simulink model "nxtway_gs"  (Simulink 10.0)
settings: Solver=ode45  StartTime=0.0  StopTime=30  MaxStep=TS  RelTol=1e-3  EnableMultiTasking=on
PreLoadFcn:
  | param_nxtway_gs
undefined symbols (not defined in the file): BATTERY, D, GP_MAX, GYRO0, MAP_WALL, pwm_gain, pwm_offset, R, sigbuilder_block, START_POS, TIME_START, W
libraries: simulink x2
settings Model: Creator=y_yama  LastModifiedBy=bhisma
settings DataIOCC: SignalLoggingSaveFormat=ModelDataLogs  SaveOutput=off  SignalLogging=off  SaveTime=off
settings OptimizationCC: DefaultParameterBehavior=Inlined  InlineInvariantSignals=on  ExpressionDepthLimit=2147483647  InitFltsAndDblsToZero=on  LifeSpan=1
settings DebuggingCC: SolverPrmCheckMsg=warning  TasksWithSamePriorityMsg=none  SigSpecEnsureSampleTimeMsg=none  IntegerOverflowMsg=none  FcnCallInpInsideContextMsg=warning  UnknownTsInhSupMsg=none  StateNameClashWarn=warning  IntegerSaturationMsg=none
settings HardwareCC: ProdLargestAtomicInteger=Long  ProdLargestAtomicFloat=Float  ProdIntDivRoundTo=Zero  ProdEndianess=LittleEndian  ProdHWDeviceType=ARM Compatible->ARM 7
settings SFSimCC: SFSimEcho=off  SimUseLocalCustomCode=on  SimParseCustomCode=off  CustomCodeUndefinedFunction=FilterOut
settings RTWCC: RTWUseLocalCustomCode=on

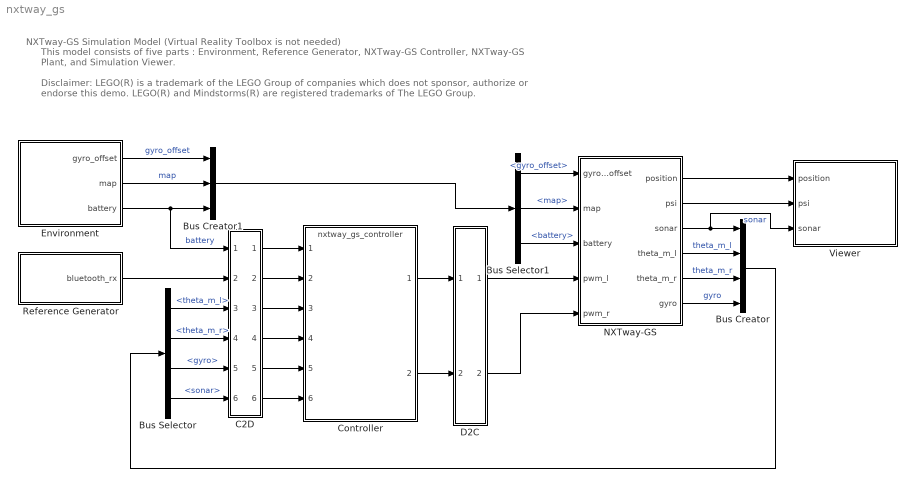
== system nxtway_gs ==
  note: Disclaimer:
      | LEGO(R) is a trademark of the LEGO Group of companies which does not sponsor, authorize or endorse this demo.
      | LEGO(R) and Mindstorms(R) are registered trademarks of The LEGO Group.
  note: NXTway-GS Simulation Model (Virtual Reality Toolbox is not needed)
  note: This model consists of five parts : Environment, Reference Generator, NXTway-GS Controller, NXTway-GS Plant, and Simulation Viewer.
  Bus Creator : BusCreator  Inputs=4
  Bus Creator1 : BusCreator  Inputs=3
  Bus Selector : BusSelector  OutputSignals=theta_m_l,theta_m_r,gyro,sonar
  Bus Selector1 : BusSelector  OutputSignals=gyro_offset,map,battery
  C2D : Subsystem
      mask Display: fprintf('C2D')
  Controller : ModelReference  ModelNameDialog=nxtway_gs_controller  SimulationMode=Normal  ModelReferenceVersion=1.721
  D2C : Subsystem
      mask Display: fprintf('D2C')
  Environment : Subsystem
  NXTway-GS : Subsystem
  Reference Generator : Subsystem
  Viewer : Subsystem
  wires:
  Bus Creator/1 -> Bus Selector/1
  Environment/3(battery) -> C2D/1(In1), Bus Creator1/3  "battery"
  Controller/1 -> D2C/1(In1)
  D2C/1(Out1) -> NXTway-GS/4(pwm_l)
  Controller/2 -> D2C/2(In2)
  D2C/2(Out2) -> NXTway-GS/5(pwm_r)
  C2D/1(Out1) -> Controller/1
  Reference Generator/1(bluetooth_rx) -> C2D/2(In2)
  C2D/2(Out2) -> Controller/2
  Bus Selector/1 -> C2D/3(In3)  "<theta_m_l>"
  Bus Selector/2 -> C2D/4(In4)  "<theta_m_r>"
  Bus Selector/3 -> C2D/5(In5)  "<gyro>"
  Bus Selector/4 -> C2D/6(In6)  "<sonar>"
  C2D/3(Out3) -> Controller/3
  C2D/4(Out4) -> Controller/4
  C2D/5(Out5) -> Controller/5
  C2D/6(Out6) -> Controller/6
  Environment/1(gyro_offset) -> Bus Creator1/1  "gyro_offset"
  Environment/2(map) -> Bus Creator1/2  "map"
  Bus Creator1/1 -> Bus Selector1/1
  Bus Selector1/1 -> NXTway-GS/1(gyro_offset)  "<gyro_offset>"
  Bus Selector1/2 -> NXTway-GS/2(map)  "<map>"
  Bus Selector1/3 -> NXTway-GS/3(battery)  "<battery>"
  NXTway-GS/2(psi) -> Viewer/2(psi)
  NXTway-GS/1(position) -> Viewer/1(position)
  NXTway-GS/3(sonar) -> Bus Creator/1, Viewer/3(sonar)  "sonar"
  NXTway-GS/4(theta_m_l) -> Bus Creator/2  "theta_m_l"
  NXTway-GS/5(theta_m_r) -> Bus Creator/3  "theta_m_r"
  NXTway-GS/6(gyro) -> Bus Creator/4  "gyro"

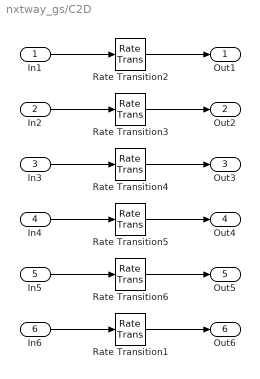
== system nxtway_gs/C2D ==
  In1 : Inport
  In2 : Inport  Port=2
  In3 : Inport  Port=3
  In4 : Inport  Port=4
  In5 : Inport  Port=5
  In6 : Inport  Port=6
  Rate Transition{1..6} (6 alike) : RateTransition  Integrity=off  OutPortSampleTime=TS
      settings: AttributesFormatString=Ts=%<OutPortSampleTime>
  Out1 : Outport
  Out2 : Outport  Port=2
  Out3 : Outport  Port=3
  Out4 : Outport  Port=4
  Out5 : Outport  Port=5
  Out6 : Outport  Port=6
  wires:
  In1/1 -> Rate Transition2/1
  Rate Transition2/1 -> Out1/1
  In2/1 -> Rate Transition3/1
  In3/1 -> Rate Transition4/1
  Rate Transition3/1 -> Out2/1
  Rate Transition4/1 -> Out3/1
  In4/1 -> Rate Transition5/1
  Rate Transition5/1 -> Out4/1
  In5/1 -> Rate Transition6/1
  Rate Transition6/1 -> Out5/1
  In6/1 -> Rate Transition1/1
  Rate Transition1/1 -> Out6/1

== system nxtway_gs/D2C ==
  In1 : Inport
  In2 : Inport  Port=2
  Rate Transition : RateTransition  Integrity=off  OutPortSampleTime=0
      settings: AttributesFormatString=Ts=%<OutPortSampleTime>
  Rate Transition1 : RateTransition  Integrity=off  OutPortSampleTime=0
      settings: AttributesFormatString=Ts=%<OutPortSampleTime>
  Out1 : Outport  SampleTime=0
  Out2 : Outport  Port=2  SampleTime=0
  wires:
  Rate Transition/1 -> Out1/1
  In1/1 -> Rate Transition/1
  Rate Transition1/1 -> Out2/1
  In2/1 -> Rate Transition1/1

== system nxtway_gs/Environment ==
  note: Environment
  note: The charactaristics of sensors of NXTway-GS and external environment.
  Constant : Constant  Value=GYRO0  OutDataTypeStr=uint16
      settings: AttributesFormatString=DataType = %<OutDataTypeStr>
  Constant1 : Constant  Value=MAP_WALL  VectorParams1D=off  OutDataTypeStr=boolean
      settings: AttributesFormatString=DataType = %<OutDataTypeStr>
  Constant2 : Constant  Value=BATTERY  OutDataTypeStr=uint16
      settings: AttributesFormatString=DataType = %<OutDataTypeStr>
  gyro_offset : Outport
  map : Outport  Port=2
  battery : Outport  Port=3
  wires:
  Constant1/1 -> map/1
  Constant/1 -> gyro_offset/1
  Constant2/1 -> battery/1

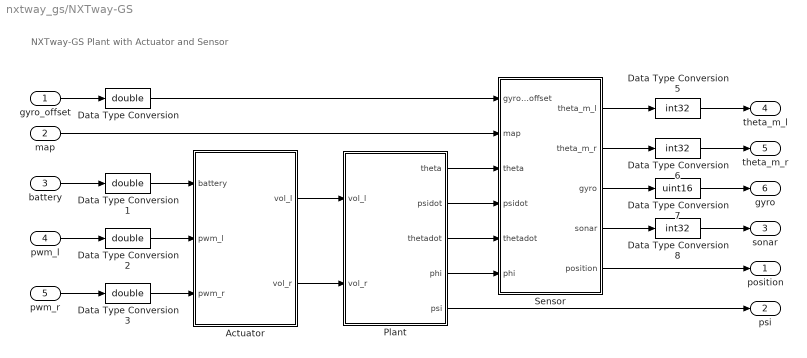
== system nxtway_gs/NXTway-GS ==
  note: NXTway-GS Plant with Actuator and Sensor
  gyro_offset : Inport
  map : Inport  Port=2
  battery : Inport  Port=3
  pwm_l : Inport  Port=4
  pwm_r : Inport  Port=5
  Actuator : Subsystem
  Data Type Conversion{,1..3} (4 alike) : DataTypeConversion  OutDataTypeStr=double  RndMeth=Nearest
      settings: AttributesFormatString=Round = %<RndMeth>
  Data Type Conversion5 : DataTypeConversion  OutDataTypeStr=int32  RndMeth=Nearest
      settings: AttributesFormatString=Round = %<RndMeth>
  Data Type Conversion6 : DataTypeConversion  OutDataTypeStr=int32  RndMeth=Nearest
      settings: AttributesFormatString=Round = %<RndMeth>
  Data Type Conversion7 : DataTypeConversion  OutDataTypeStr=uint16  RndMeth=Nearest
      settings: AttributesFormatString=Round = %<RndMeth>
  Data Type Conversion8 : DataTypeConversion  OutDataTypeStr=int32  RndMeth=Nearest
      settings: AttributesFormatString=Round = %<RndMeth>
  Plant : Subsystem
  Sensor : Subsystem
  position : Outport
  psi : Outport  Port=2
  sonar : Outport  Port=3
  theta_m_l : Outport  Port=4
  theta_m_r : Outport  Port=5
  gyro : Outport  Port=6
  wires:
  Actuator/1(vol_l) -> Plant/1(vol_l)
  Actuator/2(vol_r) -> Plant/2(vol_r)
  Plant/2(psidot) -> Sensor/4(psidot)
  Plant/1(theta) -> Sensor/3(theta)
  battery/1 -> Data Type Conversion1/1
  gyro_offset/1 -> Data Type Conversion/1
  map/1 -> Sensor/2(map)
  Sensor/1(theta_m_l) -> Data Type Conversion5/1
  Sensor/2(theta_m_r) -> Data Type Conversion6/1
  pwm_l/1 -> Data Type Conversion2/1
  Sensor/3(gyro) -> Data Type Conversion7/1
  Plant/3(thetadot) -> Sensor/5(thetadot)
  Sensor/4(sonar) -> Data Type Conversion8/1
  pwm_r/1 -> Data Type Conversion3/1
  Plant/5(psi) -> psi/1
  Data Type Conversion/1 -> Sensor/1(gyro_offset)
  Data Type Conversion1/1 -> Actuator/1(battery)
  Data Type Conversion2/1 -> Actuator/2(pwm_l)
  Data Type Conversion3/1 -> Actuator/3(pwm_r)
  Data Type Conversion5/1 -> theta_m_l/1
  Data Type Conversion6/1 -> theta_m_r/1
  Data Type Conversion7/1 -> gyro/1
  Sensor/5(position) -> position/1
  Plant/4(phi) -> Sensor/6(phi)
  Data Type Conversion8/1 -> sonar/1

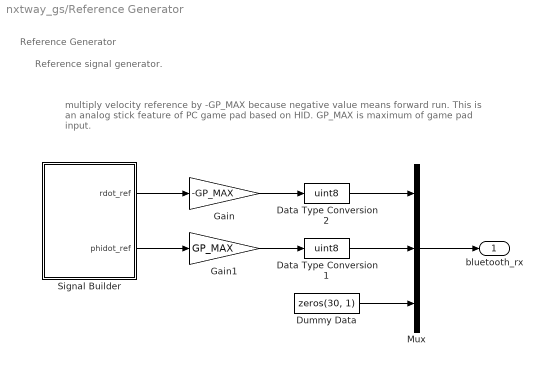
== system nxtway_gs/Reference Generator ==
  note: Reference Generator
  note: Reference signal generator.
  note: multiply velocity reference by -GP_MAX because negative value
      | means forward run. This is an analog stick feature of PC game pad
      | based on HID. GP_MAX is maximum of game pad input.
  Data Type Conversion1 : DataTypeConversion  OutDataTypeStr=uint8  RndMeth=Nearest
      settings: AttributesFormatString=Round = %<RndMeth>
  Data Type Conversion2 : DataTypeConversion  OutDataTypeStr=uint8  RndMeth=Nearest
      settings: AttributesFormatString=Round = %<RndMeth>
  Dummy Data : Constant  Value=zeros(30, 1)  OutDataTypeStr=uint8
      settings: AttributesFormatString=DataType = %<OutDataTypeStr>
  Gain : Gain  Gain=-GP_MAX  OutDataTypeStr=Inherit: Same as input  ParamDataTypeStr=Inherit: Same as input
  Gain1 : Gain  Gain=GP_MAX  OutDataTypeStr=Inherit: Same as input  ParamDataTypeStr=Inherit: Same as input
  Mux : Mux  Inputs=3
  Signal Builder : Subsystem  Tag=STV Subsys  LoadFcn=sigbuilder_block('load');  StartFcn=sigbuilder_block('start');  StopFcn=sigbuilder_block('stop');  ClipboardFcn=sigbuilder_block('clipboard');  mask(Sigbuilder block){tuvar=[0:10]}
      mask help: Sigbuilder GUI
      mask init:
      | if ~strcmp(get_param(bdroot(gcbh),'SimulationStatus'),'stopped') tuvar = sigbuilder_block('maskInit'); end
      settings: CopyFcn=sigbuilder_block('copy');  DeleteFcn=sigbuilder_block('delete');  ModelCloseFcn=sigbuilder_block('modelClose');  PreSaveFcn=sigbuilder_block('preSave');  PauseFcn=sigbuilder_block('pause')  ContinueFcn=sigbuilder_block('continue')  NameChangeFcn=sigbuilder_block('namechange');  OpenFcn=sigbuilder_block('open',[103.5 117.75 516 349.5 ]);  CloseFcn=sigbuilder_block('close');
      mask Display: plot(0, 0, 100, 100,[2, 2, 32, 32, 2], [68, 8, 8, 68, 68],[32, 2], [38, 38], [32, 19, 2],[53, 60, 44], [32, 17, 17, 2],[16, 16, 31, 31]);txt = getActiveGroup(gcbh);text(2, 100, txt,'verticalAlignment', 'top');
  bluetooth_rx : Outport
  wires:
  Data Type Conversion2/1 -> Mux/1
  Data Type Conversion1/1 -> Mux/2
  Dummy Data/1 -> Mux/3
  Mux/1 -> bluetooth_rx/1
  Signal Builder/1(rdot_ref) -> Gain/1
  Gain/1 -> Data Type Conversion2/1
  Gain1/1 -> Data Type Conversion1/1
  Signal Builder/2(phidot_ref) -> Gain1/1

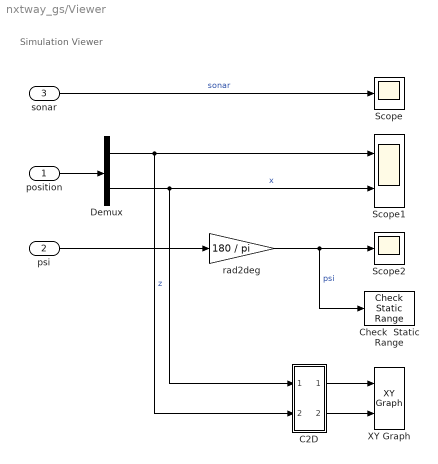
== system nxtway_gs/Viewer ==
  note: Simulation Viewer
  position : Inport
  psi : Inport  Port=2
  sonar : Inport  Port=3
  C2D : Subsystem
      mask Display: fprintf('C2D')
  Check  Static Range : simulink/Model Verification/Check  Static Range  Description=BODY_ANGLE_MIN <= u <= BODY_ANGLE_MAX  max=BODY_ANGLE_MAX  max_included=on  min=BODY_ANGLE_MIN  min_included=on  enabled=on  stopWhenAssertionFail=on  export=off  icon=graphic
      settings: SourceProductName=Simulink  SourceProductBaseCode=SL
  Demux : Demux  Outputs=2
  Scope : Scope
  Scope1 : Scope  NumInputPorts=2
  Scope2 : Scope
  XY Graph : simulink/Sinks/XY Graph  xmin=-100  xmax=300  ymin=-100  ymax=300  st=-1
  rad2deg : Gain  Gain=180 / pi
  wires:
  rad2deg/1 -> Check  Static Range/1, Scope2/1  "psi"
  Demux/1 -> Scope1/1, C2D/2(In2)  "z"
  Demux/2 -> Scope1/2, C2D/1(In1)  "x"
  psi/1 -> rad2deg/1
  sonar/1 -> Scope/1  "sonar"
  position/1 -> Demux/1
  C2D/1(Out1) -> XY Graph/1
  C2D/2(Out2) -> XY Graph/2

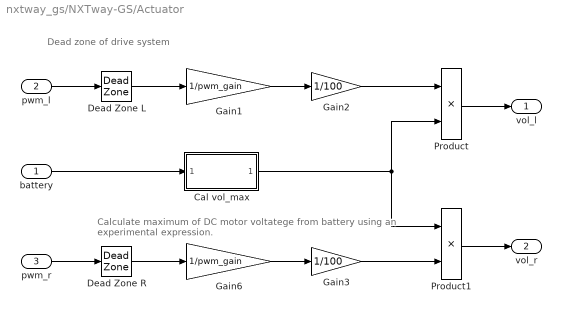
== system nxtway_gs/NXTway-GS/Actuator ==
  note: Dead zone of drive system
  note: Calculate maximum of DC motor voltatege from
      | battery using an experimental expression.
  battery : Inport
  pwm_l : Inport  Port=2
  pwm_r : Inport  Port=3
  Cal vol_max : Subsystem
  Dead Zone L : DeadZone  LowerValue=-pwm_offset  UpperValue=pwm_offset  SaturateOnIntegerOverflow=on
      settings: AttributesFormatString=start=%<LowerValue>\nend=%<UpperValue>
  Dead Zone R : DeadZone  LowerValue=-pwm_offset  UpperValue=pwm_offset  SaturateOnIntegerOverflow=on
      settings: AttributesFormatString=start=%<LowerValue>\nend=%<UpperValue>
  Gain1 : Gain  Gain=1/pwm_gain  OutDataTypeStr=Inherit: Same as input  ParamDataTypeStr=Inherit: Same as input
  Gain2 : Gain  Gain=1/100  OutDataTypeStr=Inherit: Same as input  ParamDataTypeStr=Inherit: Same as input
  Gain3 : Gain  Gain=1/100  OutDataTypeStr=Inherit: Same as input  ParamDataTypeStr=Inherit: Same as input
  Gain6 : Gain  Gain=1/pwm_gain  OutDataTypeStr=Inherit: Same as input  ParamDataTypeStr=Inherit: Same as input
  Product : Product  RndMeth=Simplest
  Product1 : Product  RndMeth=Simplest
  vol_l : Outport
  vol_r : Outport  Port=2
  wires:
  pwm_l/1 -> Dead Zone L/1
  pwm_r/1 -> Dead Zone R/1
  Gain1/1 -> Gain2/1
  Gain6/1 -> Gain3/1
  Gain2/1 -> Product/1
  Product/1 -> vol_l/1
  Gain3/1 -> Product1/2
  Product1/1 -> vol_r/1
  Dead Zone L/1 -> Gain1/1
  Dead Zone R/1 -> Gain6/1
  Cal vol_max/1(vol_max) -> Product/2, Product1/1
  battery/1 -> Cal vol_max/1(battery)

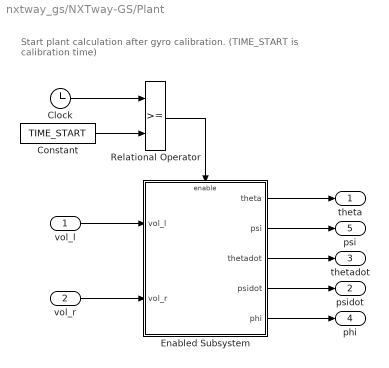
== system nxtway_gs/NXTway-GS/Plant ==
  note: Start plant calculation after gyro calibration.
      | (TIME_START is calibration time)
  vol_l : Inport
  vol_r : Inport  Port=2
  Clock : Clock
  Constant : Constant  Value=TIME_START  OutDataTypeStr=double
      settings: AttributesFormatString=DataType = %<OutDataTypeStr>
  Enabled Subsystem : Subsystem  TreatAsAtomicUnit=on
  Relational Operator : RelationalOperator  OutDataTypeStr=boolean  RndMeth=Nearest
  theta : Outport
  psidot : Outport  Port=2
  thetadot : Outport  Port=3
  phi : Outport  Port=4
  psi : Outport  Port=5
  wires:
  vol_l/1 -> Enabled Subsystem/1(vol_l)
  vol_r/1 -> Enabled Subsystem/2(vol_r)
  Relational Operator/1 -> Enabled Subsystem/Enable
  Clock/1 -> Relational Operator/1
  Constant/1 -> Relational Operator/2
  Enabled Subsystem/1(theta) -> theta/1
  Enabled Subsystem/3(thetadot) -> thetadot/1
  Enabled Subsystem/2(psi) -> psi/1
  Enabled Subsystem/5(phi) -> phi/1
  Enabled Subsystem/4(psidot) -> psidot/1

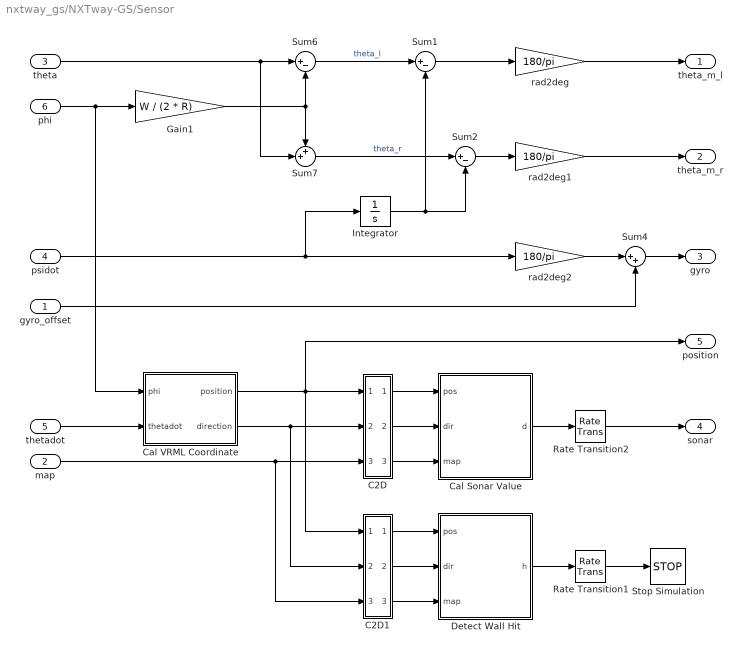
== system nxtway_gs/NXTway-GS/Sensor ==
  gyro_offset : Inport
  map : Inport  Port=2
  theta : Inport  Port=3
  psidot : Inport  Port=4
  thetadot : Inport  Port=5
  phi : Inport  Port=6
  C2D : Subsystem
      mask Display: fprintf('C2D')
  C2D1 : Subsystem
      mask Display: fprintf('C2D')
  Cal Sonar Value : MATLAB Function  TreatAsAtomicUnit=on
  Cal VRML Coordinate : Subsystem
  Detect Wall Hit : MATLAB Function  TreatAsAtomicUnit=on
  Gain1 : Gain  Gain=W / (2 * R)
  Integrator : Integrator
  Rate Transition1 : RateTransition  Integrity=off  OutPortSampleTime=0
      settings: AttributesFormatString=Ts=%<OutPortSampleTime>
  Rate Transition2 : RateTransition  Integrity=off  OutPortSampleTime=0
      settings: AttributesFormatString=Ts=%<OutPortSampleTime>
  Stop Simulation : Stop
  Sum1 : Sum  Inputs=|+-
  Sum2 : Sum  Inputs=|+-
  Sum4 : Sum  Inputs=|++
  Sum6 : Sum  Inputs=|+-
  Sum7 : Sum  Inputs=++|
  rad2deg : Gain  Gain=180/pi
  rad2deg1 : Gain  Gain=180/pi
  rad2deg2 : Gain  Gain=180/pi
  theta_m_l : Outport
  theta_m_r : Outport  Port=2
  gyro : Outport  Port=3
  sonar : Outport  Port=4
  position : Outport  Port=5
  wires:
  Integrator/1 -> Sum2/2, Sum1/2
  Sum4/1 -> gyro/1
  gyro_offset/1 -> Sum4/2
  Sum7/1 -> Sum2/1  "theta_r"
  rad2deg2/1 -> Sum4/1
  theta/1 -> Sum7/2, Sum6/1
  phi/1 -> Gain1/1, Cal VRML Coordinate/1(phi)
  Gain1/1 -> Sum7/1, Sum6/2
  Sum1/1 -> rad2deg/1
  psidot/1 -> Integrator/1, rad2deg2/1
  Sum2/1 -> rad2deg1/1
  rad2deg/1 -> theta_m_l/1
  rad2deg1/1 -> theta_m_r/1
  Sum6/1 -> Sum1/1  "theta_l"
  thetadot/1 -> Cal VRML Coordinate/2(thetadot)
  Cal Sonar Value/1(d) -> Rate Transition2/1
  Rate Transition2/1 -> sonar/1
  Cal VRML Coordinate/1(position) -> position/1, C2D/1(In1), C2D1/1(In1)
  map/1 -> C2D1/3(In3), C2D/3(In3)
  C2D/3(Out3) -> Cal Sonar Value/3(map)
  C2D/1(Out1) -> Cal Sonar Value/1(pos)
  Cal VRML Coordinate/2(direction) -> C2D/2(In2), C2D1/2(In2)
  C2D/2(Out2) -> Cal Sonar Value/2(dir)
  Detect Wall Hit/1(h) -> Rate Transition1/1
  C2D1/1(Out1) -> Detect Wall Hit/1(pos)
  C2D1/2(Out2) -> Detect Wall Hit/2(dir)
  C2D1/3(Out3) -> Detect Wall Hit/3(map)
  Rate Transition1/1 -> Stop Simulation/1

== system nxtway_gs/Reference Generator/Signal Builder ==
  Demux : Demux  Tag=STV Demux  Outputs=2
  FromWs : FromWorkspace  Tag=STV FromWs  VariableName=tuvar  SampleTime=0  SigBuilderData=DataTag0  VnvData=DataTag1
      SigBuilderData=|
      | common.afterFinalStr = 'Extrapolate'
      | common.sampleTime = 0
      | dataSet(1).timeRange = [0 25]
      | dataSet(1).name = 'Stand'
      | dataSet(2).timeRange = [0 25]
      | dataSet(2).name = 'Forward & Back'
      | dataSet(3).timeRange = [0 25]
      | dataSet(3).name = 'Turn'
      | dataSet(4).timeRange = [0 25]
      | dataSet(4).name = 'Approach Wall'
      | sbobj.Groups(1).Name = 'Stand'
      | sbobj.Groups(1).Signals(1).Name = 'rdot_ref'
      | sbobj.Groups(1).Signals(1).XData = [0 25]
      | sbobj.Groups(1).Signals(1).YData = [0 0]
      | sbobj.Groups(1).Signals(2).Name = 'phidot_ref'
      | sbobj.Groups(1).Signals(2).XData = [0 25]
      | sbobj.Groups(1).Signals(2).YData = [0 0]
      | sbobj.Groups(1).TimeRange = [0 25]
      | sbobj.Groups(2).Name = 'Forward & Back'
      | sbobj.Groups(2).Signals(1).Name = 'rdot_ref'
      | sbobj.Groups(2).Signals(1).XData = [0 5 5 10 10 15 15 20 20 25]
      | sbobj.Groups(2).Signals(1).YData = [0 0 1 1 0 0 -1 -1 0 0]
      | sbobj.Groups(2).Signals(2).Name = 'phidot_ref'
      | sbobj.Groups(2).Signals(2).XData = [0 25]
      | sbobj.Groups(2).Signals(2).YData = [0 0]
      | sbobj.Groups(2).TimeRange = [0 25]
      | sbobj.Groups(3).Name = 'Turn'
      | sbobj.Groups(3).Signals(1).Name = 'rdot_ref'
      | sbobj.Groups(3).Signals(1).XData = [0 10 10 15 15 20 20 25]
      | sbobj.Groups(3).Signals(1).YData = [0 0 1 1 0 0 1 1]
      | sbobj.Groups(3).Signals(2).Name = 'phidot_ref'
      | sbobj.Groups(3).Signals(2).XData = [0 5 5 10 10 15 15 20 20 25]
      | sbobj.Groups(3).Signals(2).YData = [0 0 1 1 0 0 -1 -1 0 0]
      | sbobj.Groups(3).TimeRange = [0 25]
      | sbobj.Groups(4).Name = 'Approach Wall'
      | sbobj.Groups(4).Signals(1).Name = 'rdot_ref'
      | sbobj.Groups(4).Signals(1).XData = [0 6.4 6.4 25]
      | sbobj.Groups(4).Signals(1).YData = [0 0 1 1]
      | sbobj.Groups(4).Signals(2).Name = 'phidot_ref'
      | sbobj.Groups(4).Signals(2).XData = [0 5 5 6.4 6.4 15 20 25]
      | sbobj.Groups(4).Signals(2).YData = [0 0 -1 -1 0 0 0 0]
      | sbobj.Groups(4).TimeRange = [0 25]
  rdot_ref : Outport  Tag=STV Outport
  phidot_ref : Outport  Tag=STV Outport  Port=2
  wires:
  FromWs/1 -> Demux/1
  Demux/1 -> rdot_ref/1
  Demux/2 -> phidot_ref/1

== system nxtway_gs/Viewer/C2D ==
  In1 : Inport
  In2 : Inport  Port=2
  Rate Transition1 : RateTransition  Integrity=off  OutPortSampleTime=TS_VR
      settings: AttributesFormatString=Ts=%<OutPortSampleTime>
  Rate Transition2 : RateTransition  Integrity=off  OutPortSampleTime=TS_VR
      settings: AttributesFormatString=Ts=%<OutPortSampleTime>
  Out1 : Outport
  Out2 : Outport  Port=2
  wires:
  Rate Transition1/1 -> Out2/1
  In2/1 -> Rate Transition1/1
  Rate Transition2/1 -> Out1/1
  In1/1 -> Rate Transition2/1

== system nxtway_gs/NXTway-GS/Actuator/Cal vol_max ==
  battery : Inport
  Constant : Constant  Value=0.625  OutDataTypeStr=double
      settings: AttributesFormatString=DataType = %<OutDataTypeStr>
  Gain3 : Gain  Gain=0.001089  OutDataTypeStr=Inherit: Same as input  ParamDataTypeStr=Inherit: Same as input
  Sum2 : Sum  Inputs=|+-  OutDataTypeStr=Inherit: Same as first input
  vol_max : Outport
  wires:
  battery/1 -> Gain3/1
  Gain3/1 -> Sum2/1
  Sum2/1 -> vol_max/1
  Constant/1 -> Sum2/2

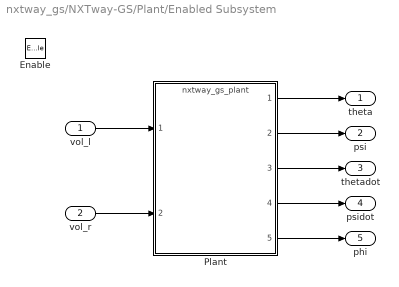
== system nxtway_gs/NXTway-GS/Plant/Enabled Subsystem ==
  vol_l : Inport
  vol_r : Inport  Port=2
  Enable : EnablePort
  Plant : ModelReference  ModelNameDialog=nxtway_gs_plant  SimulationMode=Normal  ModelReferenceVersion=1.41
  theta : Outport  InitialOutput=0
  psi : Outport  Port=2  InitialOutput=0
  thetadot : Outport  Port=3  InitialOutput=0
  psidot : Outport  Port=4  InitialOutput=0
  phi : Outport  Port=5  InitialOutput=0
  wires:
  vol_l/1 -> Plant/1
  vol_r/1 -> Plant/2
  Plant/1 -> theta/1
  Plant/2 -> psi/1
  Plant/3 -> thetadot/1
  Plant/4 -> psidot/1
  Plant/5 -> phi/1

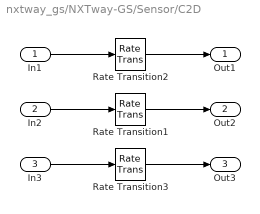
== system nxtway_gs/NXTway-GS/Sensor/C2D ==
  In1 : Inport
  In2 : Inport  Port=2
  In3 : Inport  Port=3
  Rate Transition1 : RateTransition  Integrity=off  OutPortSampleTime=TS_SONAR
      settings: AttributesFormatString=Ts=%<OutPortSampleTime>
  Rate Transition2 : RateTransition  Integrity=off  OutPortSampleTime=TS_SONAR
      settings: AttributesFormatString=Ts=%<OutPortSampleTime>
  Rate Transition3 : RateTransition  Integrity=off  OutPortSampleTime=TS_SONAR
      settings: AttributesFormatString=Ts=%<OutPortSampleTime>
  Out1 : Outport
  Out2 : Outport  Port=2
  Out3 : Outport  Port=3
  wires:
  Rate Transition3/1 -> Out3/1
  Rate Transition1/1 -> Out2/1
  In3/1 -> Rate Transition3/1
  In2/1 -> Rate Transition1/1
  Rate Transition2/1 -> Out1/1
  In1/1 -> Rate Transition2/1

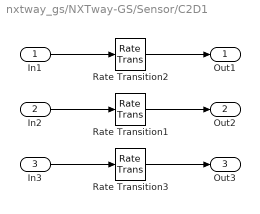
== system nxtway_gs/NXTway-GS/Sensor/C2D1 ==
  In1 : Inport
  In2 : Inport  Port=2
  In3 : Inport  Port=3
  Rate Transition1 : RateTransition  Integrity=off  OutPortSampleTime=TS_WALL
      settings: AttributesFormatString=Ts=%<OutPortSampleTime>
  Rate Transition2 : RateTransition  Integrity=off  OutPortSampleTime=TS_WALL
      settings: AttributesFormatString=Ts=%<OutPortSampleTime>
  Rate Transition3 : RateTransition  Integrity=off  OutPortSampleTime=TS_WALL
      settings: AttributesFormatString=Ts=%<OutPortSampleTime>
  Out1 : Outport
  Out2 : Outport  Port=2
  Out3 : Outport  Port=3
  wires:
  In1/1 -> Rate Transition2/1
  Rate Transition2/1 -> Out1/1
  In2/1 -> Rate Transition1/1
  In3/1 -> Rate Transition3/1
  Rate Transition1/1 -> Out2/1
  Rate Transition3/1 -> Out3/1

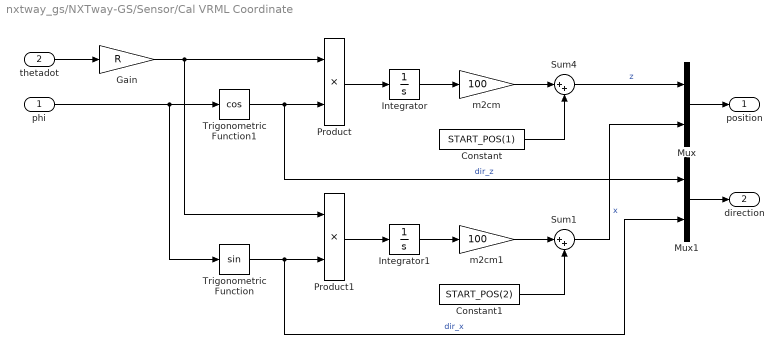
== system nxtway_gs/NXTway-GS/Sensor/Cal VRML Coordinate ==
  phi : Inport
  thetadot : Inport  Port=2
  Constant : Constant  Value=START_POS(1)  OutDataTypeStr=double
      settings: AttributesFormatString=DataType = %<OutDataTypeStr>
  Constant1 : Constant  Value=START_POS(2)  OutDataTypeStr=double
      settings: AttributesFormatString=DataType = %<OutDataTypeStr>
  Gain : Gain  Gain=R
  Integrator : Integrator
  Integrator1 : Integrator
  Mux : Mux  Inputs=2
  Mux1 : Mux  Inputs=2
  Product : Product  RndMeth=Simplest
  Product1 : Product  RndMeth=Simplest
  Sum1 : Sum  Inputs=|++
  Sum4 : Sum  Inputs=|++
  Trigonometric Function : Trigonometry
  Trigonometric Function1 : Trigonometry  Operator=cos
  m2cm : Gain  Gain=100
  m2cm1 : Gain  Gain=100
  position : Outport
  direction : Outport  Port=2
  wires:
  Product1/1 -> Integrator1/1
  Trigonometric Function/1 -> Product1/2, Mux1/2  "dir_x"
  Product/1 -> Integrator/1
  Trigonometric Function1/1 -> Product/2, Mux1/1  "dir_z"
  thetadot/1 -> Gain/1
  phi/1 -> Trigonometric Function1/1, Trigonometric Function/1
  Integrator/1 -> m2cm/1
  Integrator1/1 -> m2cm1/1
  Gain/1 -> Product1/1, Product/1
  m2cm/1 -> Sum4/1
  Sum4/1 -> Mux/1  "z"
  Constant/1 -> Sum4/2
  m2cm1/1 -> Sum1/1
  Constant1/1 -> Sum1/2
  Sum1/1 -> Mux/2  "x"
  Mux/1 -> position/1
  Mux1/1 -> direction/1

== matlab function NXTway-GS/Sensor/Detect Wall Hit ==
  data: pos input double; h output boolean; dir input double; map input double; D parameter double; W parameter double
function h = hit_wall(pos, dir, map, D, W)
% Detect if NXTway hits the wall
% Inputs:
%   pos    : NXTway position ([z, x]) [cm]
%   dir    : NXTway direction vector ([z, x]) [cm]
%   map    : wall map
% Outputs:
%   h      : wall hit flag

eml.extrinsic('errordlg');

h = false;
posh = zeros(6, 2);
[rows, cols] = size(map);
tmp1 = (D / 2) * dir;
tmp2 = (W / 2) * [dir(2), -dir(1)];

posh(2, :) = pos + tmp1;
posh(5, :) = pos - tmp1;
posh(1, :) = posh(2, :) + tmp2;
posh(6, :) = posh(5, :) + tmp2;
posh(3, :) = posh(2, :) - tmp2;
posh(4, :) = posh(5, :) - tmp2;

for n = 1:6
	if posh(n, 1) <= 0 || posh(n, 1) >= rows ...
			|| posh(n, 2) <= 0 || posh(n, 2) >= cols
		% outside map
		h = false;
	else
		% inside map
		h = iswall(posh(n, :), map);
		if h == true
			errordlg('NXTway-GS Hits Wall !', 'Wall Hit Detection');
			break;
		end
	end
end

== matlab function NXTway-GS/Sensor/Cal Sonar Value ==
  data: pos input double; dir input double; d output int32; map input double
function d = cal_sonar(pos, dir, map)
% Calcurate sonar value (distance)
% Inputs:
%   pos    : NXTway position ([z, x]) [cm]
%   dir    : NXTway direction vector ([z, x]) [cm]
%   map    : wall map
% Outputs:
%   d      : sonar value (distance) [cm]

d = 1;
[rows, cols] = size(map);

while d < 255
	posd = pos + d * dir;
	if posd(1) <= 0 || posd(1) >= rows ...
			|| posd(2) <= 0 || posd(2) >= cols
		% outside map
		d = 255;
	else
		% inside map
		flag = iswall(posd, map);
		if flag == true
			break;
		else
			d = d + 1;
		end
	end
end
